simulink model "rcModelSimulink"  (R2023a)
settings: Solver=VariableStepAuto  StartTime=0.0  StopTime=102800  RelTol=1e-3
values from neighbouring files (symbols this model uses):
  c1 = 50    [hppcModelParams.m]    (also in rcModel.m = 12)
  c2 = 40    [hppcModelParams.m]    (also in rcModel.m = 10)
  cell = struct    [cell_PANA18650PF.m]
  ocv = interp1(vSoc, vOcv, soc(t), "linear")    [endOfChargeHeatup.m]    (also in rcModelMock.m = 3)
  r0 = 0.02    [hppcModelParams.m]    (also in rcModelMock.m = 0.01)
  r1 = 0.01    [hppcModelParams.m]    (also in rcModel.m = 10)
  r2 = 0.003    [hppcModelParams.m]    (also in rcModel.m = 5)
  soc = []    [endOfChargeHeatup.m]
settings Model: Creator=deshm  LastModifiedBy=deshm

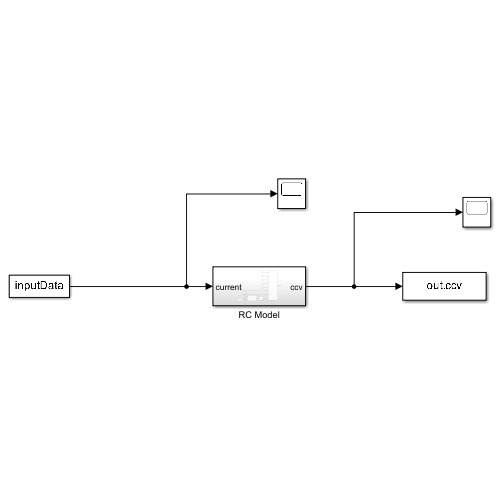
[thumbnail: Simulink's stored preview of the top-level diagram]
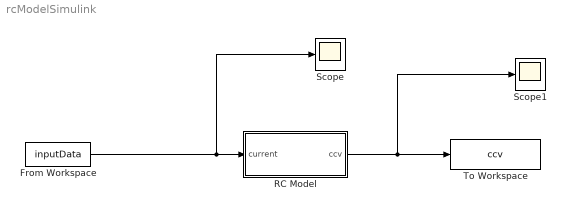
== system rcModelSimulink ==
  From Workspace : FromWorkspace  VariableName=inputData  SampleTime=0.1  OutputAfterFinalValue=Holding final value
  RC Model : Subsystem
  Scope : Scope
  Scope1 : Scope
  To Workspace : ToWorkspace  VariableName=ccv  SaveFormat=Timeseries  SampleTime=-1
  wires:
  From Workspace/1 -> Scope/1, RC Model/1(current)
  RC Model/1(ccv) -> Scope1/1, To Workspace/1

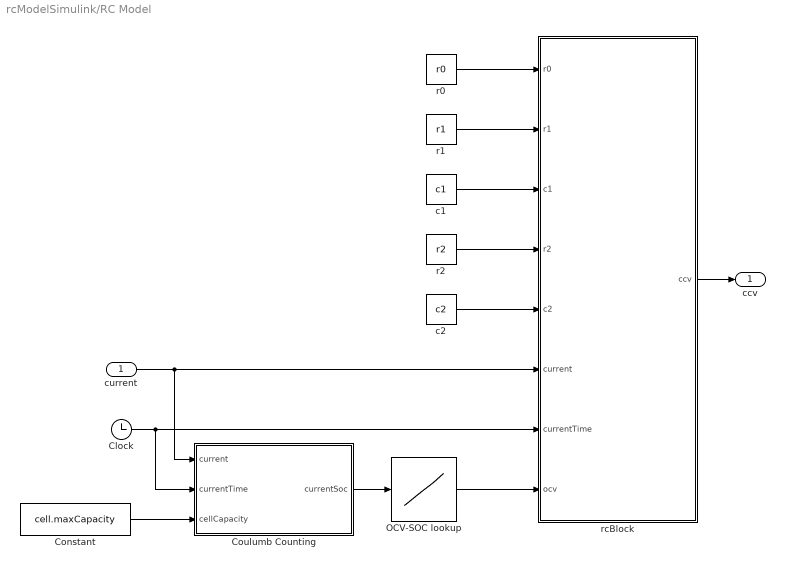
== system rcModelSimulink/RC Model ==
  current : Inport
  Clock : Clock
  Constant : Constant  Value=cell.maxCapacity
  Coulumb Counting : MATLAB Function  TreatAsAtomicUnit=on
  OCV-SOC lookup : Lookup_n-D  NumberOfTableDimensions=1  BreakpointsForDimension1=soc  Table=ocv  InternalRulePriority=Speed  RndMeth=Simplest
  c1 : Constant  Value=c1
  c2 : Constant  Value=c2
  r0 : Constant  Value=r0
  r1 : Constant  Value=r1
  r2 : Constant  Value=r2
  rcBlock : MATLAB Function  TreatAsAtomicUnit=on
  ccv : Outport
  wires:
  Coulumb Counting/1(currentSoc) -> OCV-SOC lookup/1
  Clock/1 -> rcBlock/7(currentTime), Coulumb Counting/2(currentTime)
  current/1 -> rcBlock/6(current), Coulumb Counting/1(current)
  Constant/1 -> Coulumb Counting/3(cellCapacity)
  r2/1 -> rcBlock/4(r2)
  r1/1 -> rcBlock/2(r1)
  r0/1 -> rcBlock/1(r0)
  c1/1 -> rcBlock/3(c1)
  c2/1 -> rcBlock/5(c2)
  OCV-SOC lookup/1 -> rcBlock/8(ocv)
  rcBlock/1(ccv) -> ccv/1

== matlab function rcModelSimulink/RC Model/Coulumb Counting ==
  data: current input; currentSoc output; currentTime input; cellCapacity input
function currentSoc = fcn(current, currentTime, cellCapacity)
    persistent soc
    persistent dt
    persistent previousTime

    if isempty(soc)
        soc = 100;
        previousTime = currentTime;
        dt = 0.1;
    else
        dt = currentTime - previousTime;
        previousTime = currentTime;
    end
    
    currentSoc = soc + dt * current * 100 / (cellCapacity * 3600);
    soc = currentSoc;
    
  
end

== matlab function rcModelSimulink/RC Model/rcBlock ==
  data: r0 input; ccv output; r1 input; c1 input; r2 input; c2 input; current input; currentTime input; ocv input
function ccv = fcn(r0, r1, c1, r2, c2, current, currentTime, ocv)
    persistent previousTime
    persistent vP
    
    if isempty(previousTime)
        vP = [0 0];
        previousTime = currentTime;
        dt = 0.1;
    else
        dt = currentTime - previousTime;
        previousTime = currentTime;
    end

    [ccv, vP] = rcModelForParamEstimation(ocv, current, r0, r1, c1, r2, c2, dt, vP);

end
